simulink model "simulink_caso2"  (R2023a)
settings: Solver=VariableStepAuto  StartTime=0.0  StopTime=10.0  RelTol=1e-3
undefined symbols (not defined in the file): A, Aest, B, Best, C, Cest, D, Dest, K, K0
libraries: simulink x1
settings Model: Creator=Agustin  LastModifiedBy=Agustin

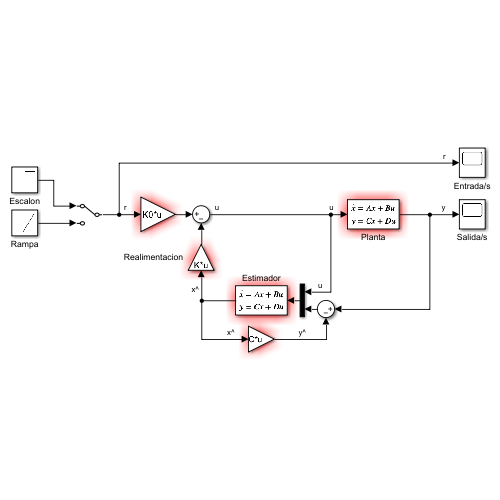
[thumbnail: Simulink's stored preview of the top-level diagram]
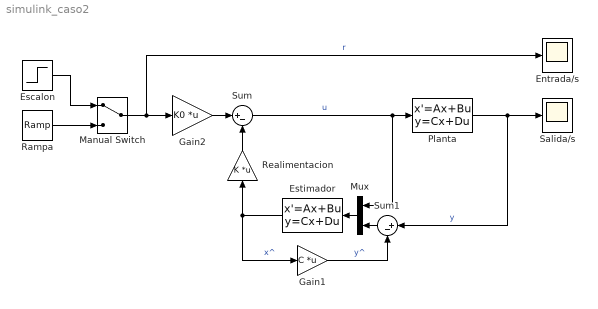
== system simulink_caso2 ==
  Entrada/s : Scope
  Escalon : Step  SampleTime=0
  Estimador : StateSpace  A=Aest  B=Best  C=Cest  D=Dest  InitialCondition=0
  Gain1 : Gain  Gain=C  Multiplication=Matrix(K*u)
  Gain2 : Gain  Gain=K0  Multiplication=Matrix(K*u)
  Manual Switch : ManualSwitch
  Mux : Mux  Inputs=2
  Planta : StateSpace  A=A  B=B  C=C  D=D  InitialCondition=0
  Rampa : simulink/Sources/Ramp  slope=1  start=0  InitialOutput=0
  Realimentacion : Gain  Gain=K  Multiplication=Matrix(K*u)
  Salida/s : Scope
  Sum : Sum  Inputs=|+-
  Sum1 : Sum  Inputs=|+-
  wires:
  Estimador/1 -> Realimentacion/1, Gain1/1  "x^"
  Realimentacion/1 -> Sum/2
  Sum/1 -> Planta/1, Mux/1  "u"
  Planta/1 -> Salida/s/1, Sum1/1  "y"
  Manual Switch/1 -> Entrada/s/1, Gain2/1  "r"
  Mux/1 -> Estimador/1
  Sum1/1 -> Mux/2
  Gain2/1 -> Sum/1
  Rampa/1 -> Manual Switch/2
  Escalon/1 -> Manual Switch/1
  Gain1/1 -> Sum1/2  "y^"
